simulink model "ch6q2"  (R2019a)
settings: Solver=VariableStepAuto  StartTime=0.0  StopTime=20  RelTol=1e-3
libraries: simulink_extras x4
settings Model: Creator=Administrator  LastModifiedBy=Administrator
settings OptimizationCC: BooleanDataType=off

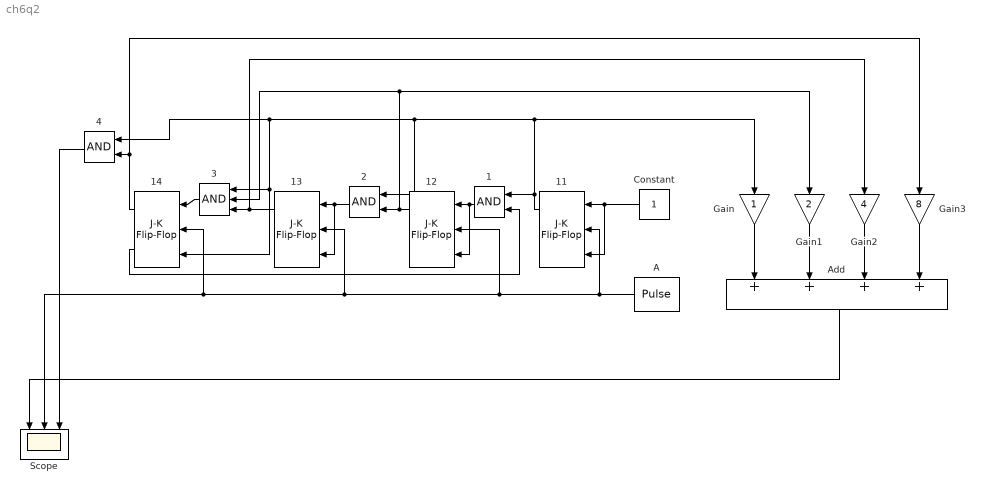
== system ch6q2 ==
  1 : Logic
  {11..14} (4 alike) : simulink_extras/Flip Flops/J-K Flip-Flop  initial_condition=0
      settings: SourceProductName=Simulink
  2 : Logic
  3 : Logic  Inputs=3
  4 : Logic  AllPortsSameDT=off  OutDataTypeStr=boolean
  A : DiscretePulseGenerator  PhaseDelay=1
  Add : Sum  Inputs=++++
  Constant : Constant  OutDataTypeStr=double
  Gain : Gain
  Gain1 : Gain  Gain=2
  Gain2 : Gain  Gain=4
  Gain3 : Gain  Gain=8
  Scope : Scope  NumInputPorts=3
  wires:
  13/1 -> Gain2/1, 3/3
  Constant/1 -> 11/3, 11/1
  14/2 -> 1/2
  12/1 -> Gain1/1, 3/2, 2/2
  1/1 -> 12/3, 12/1
  2/1 -> 13/3, 13/1
  4/1 -> Scope/3
  11/1 -> 1/1, Gain/1, 14/3, 3/1, 4/1, 2/1
  A/1 -> 11/2, 12/2, 13/2, Scope/2, 14/2
  14/1 -> Gain3/1, 4/2
  3/1 -> 14/1
  Gain2/1 -> Add/3
  Gain/1 -> Add/1
  Gain3/1 -> Add/4
  Gain1/1 -> Add/2
  Add/1 -> Scope/1
